simulink model "Actuators"  (R2021a)
settings: Solver=FixedStepAuto  StartTime=0.0  StopTime=10.0  RelTol=1e-3
undefined symbols (not defined in the file): servo
libraries: cstblocks x5
settings Model: Creator=User01  LastModifiedBy=User01

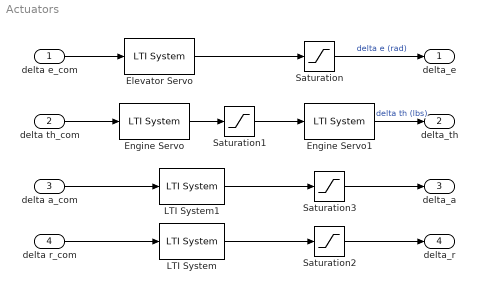
== system Actuators ==
  delta e_com : Inport
  delta th_com : Inport  Port=2
  delta a_com : Inport  Port=3
  delta r_com : Inport  Port=4
  Elevator Servo : cstblocks/LTI System  sys=-servo  IC=[]
  Engine Servo : cstblocks/LTI System  sys=servo  IC=[]
  Engine Servo1 : cstblocks/LTI System  sys=engine_timelag  IC=[]
  LTI System : cstblocks/LTI System  sys=servo  IC=[]
  LTI System1 : cstblocks/LTI System  sys=servo  IC=[]
  Saturation : Saturate  UpperLimit=25*pi/180  LowerLimit=-25*pi/180
  Saturation1 : Saturate  UpperLimit=47000  LowerLimit=-3*47000
  Saturation2 : Saturate  UpperLimit=15*pi/180  LowerLimit=-15*pi/180
  Saturation3 : Saturate  UpperLimit=50*pi/180  LowerLimit=-50*pi/180
  delta_e : Outport
  delta_th : Outport  Port=2
  delta_a : Outport  Port=3
  delta_r : Outport  Port=4
  wires:
  delta e_com/1 -> Elevator Servo/1
  Engine Servo1/1 -> delta_th/1  "delta th (lbs)"
  Saturation1/1 -> Engine Servo1/1
  Elevator Servo/1 -> Saturation/1
  Engine Servo/1 -> Saturation1/1
  Saturation/1 -> delta_e/1  "delta e (rad)"
  delta th_com/1 -> Engine Servo/1
  Saturation3/1 -> delta_a/1
  delta r_com/1 -> LTI System/1
  LTI System1/1 -> Saturation3/1
  delta a_com/1 -> LTI System1/1
  Saturation2/1 -> delta_r/1
  LTI System/1 -> Saturation2/1
